simulink model "sim_reg_posture_final"  (R2025b)
settings: Solver=VariableStepAuto  StartTime=0.0  StopTime=10  RelTol=1e-3
undefined symbols (not defined in the file): setpoints, sim_trajectory_id, Ts
settings Model: Creator=Utente  LastModifiedBy=Utente

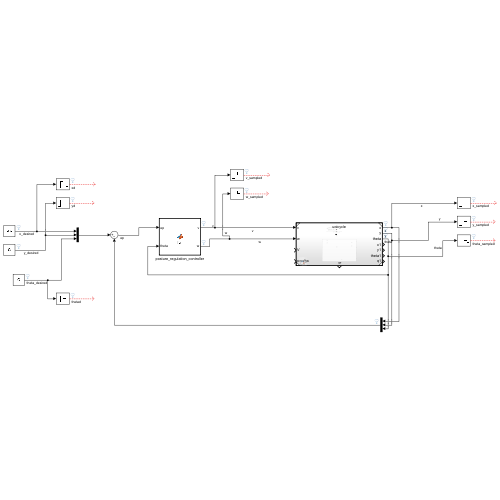
[thumbnail: Simulink's stored preview of the top-level diagram]
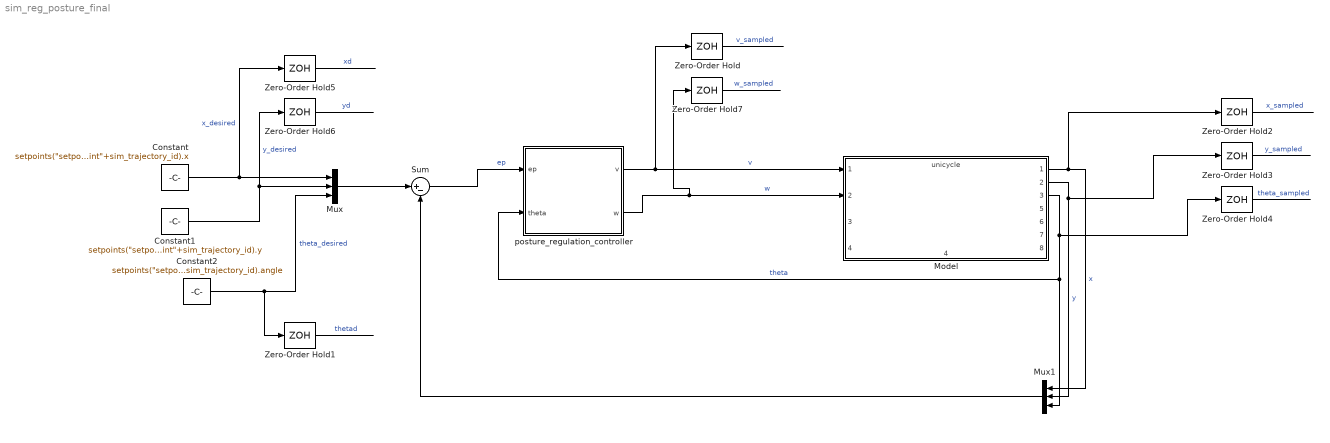
== system sim_reg_posture_final ==
  Constant : Constant  Value="setpoints(\"setpoint\"+sim_trajectory_id).x"
  Constant1 : Constant  Value="setpoints(\"setpoint\"+sim_trajectory_id).y"
  Constant2 : Constant  Value="setpoints(\"setpoint\"+sim_trajectory_id).angle"
  Model : ModelReference  ModelNameDialog=unicycle.slx  SimulationMode=Normal  ModelReferenceVersion=1.12
      settings: PortSchema="{\"entries\":[{\"content\":{\"sides\":[{\"content\":{\"connectorIds\":[\"In1\",\"In2\",\"In3\",\"In4\"]},\"type\":\"ConnectorPlacement.EquallySpacedRectSide\",\"uuid\":\"ad25d81c-9301-4260-b0e7-6964e2a4144d\"},{\"content\":{\"connectorIds\":[\"Out1\",\"Out2\",\"Out3\",\"Out5\",\"Out6\",\"Out7\",\"Out8\"],\"side\":\"RIGHT\"},\"type\":\"ConnectorPlacement.EquallySpacedRectSide\",\"uuid\":\"e119e278-1a19-4d21-ac57-f30b4b2846c4\"},{\"content\":{\"side\":\"TOP\"},\"type\":\"ConnectorPlacement.EquallySpacedRectSide\",\"uuid\":\"f58ebd06-2844-4b35-9f44-2944c544d228\"},{\"content\":{\"connectorIds\":[\"Out4\"],\"side\":\"BOTTOM\"},\"type\":\"ConnectorPlacement.EquallySpacedRectSide\",\"uuid\":\"e9666c6b-2f60-424a-96df-bac3fd1a20e8\"}]},\"type\":\"ConnectorPlacement.EquallySpacedConnector\",\"uuid\":\"feeb8aec-4c5e-4f88-9f0a-836c4fc89b7c\"}],\"packageUris\":[\"http://schema.mathworks.com/mf0/Connector/R2020b\"],\"version\":\"1.0\"}"
  Mux : Mux  Inputs=3
  Mux1 : Mux  Inputs=3
  Sum : Sum  Inputs=|+-
  Zero-Order Hold{,1..7} (8 alike) : ZeroOrderHold  SampleTime=Ts
  posture_regulation_controller : MATLAB Function  TreatAsAtomicUnit=on
  wires:
  Mux1/1 -> Sum/2
  Constant/1 -> Zero-Order Hold5/1, Mux/1  "x_desired"
  Constant1/1 -> Zero-Order Hold6/1, Mux/2  "y_desired"
  Mux/1 -> Sum/1
  Constant2/1 -> Zero-Order Hold1/1, Mux/3  "theta_desired"
  Sum/1 -> posture_regulation_controller/1(ep)  "ep"
  Zero-Order Hold5/1 -> ?  "xd"
  Zero-Order Hold6/1 -> ?  "yd"
  Zero-Order Hold1/1 -> ?  "thetad"
  Model/1 -> Zero-Order Hold2/1, Mux1/1  "x"
  Model/3 -> Zero-Order Hold4/1, Mux1/3, posture_regulation_controller/2(theta)  "theta"
  Zero-Order Hold2/1 -> ?  "x_sampled"
  Model/2 -> Zero-Order Hold3/1, Mux1/2  "y"
  Zero-Order Hold4/1 -> ?  "theta_sampled"
  Zero-Order Hold3/1 -> ?  "y_sampled"
  Zero-Order Hold/1 -> ?  "v_sampled"
  Zero-Order Hold7/1 -> ?  "w_sampled"
  posture_regulation_controller/2(w) -> Zero-Order Hold7/1, Model/2  "w"
  posture_regulation_controller/1(v) -> Zero-Order Hold/1, Model/1  "v"

== matlab function sim_reg_posture_final/posture_regulation_controller ==
  data: ep input; v output; w output; theta input
function [v, w] = fcn(ep, theta)

dx = ep(1);
dy = ep(2);
dtheta = -ep(3);

rho   = sqrt(dx^2 + dy^2);
%alpha = wrapToPi(atan2(dy, dx) - theta); 
%beta  = wrapToPi(dtheta - alpha);
gamma = wrapToPi(atan2(dy, dx) - theta);
delta = wrapToPi(dtheta - gamma);

k1 = 1;%1
k2 = 4;%4
k3 = 1.5;%1.5

v = k1 * rho * cos(gamma);
w = k2 * gamma + k1 * sin(gamma) * cos(gamma)/gamma * (gamma+k3*delta);

end
